simulink model "NL_sin_Park_funciona"  (R2023b)
settings: Solver=VariableStepAuto  StartTime=0.0  StopTime=2  MaxStep=1e-3  RelTol=1e-3
values from neighbouring files (symbols this model uses):
  alpha_Cu = 3.9e-3    (= 0.0039)    [definicion_cte.m]
  b_eq = b_m + b_l/(r^2)    (= 2.40277777778e-05)    [definicion_cte.m]
  C_ts = 0.818    [definicion_cte.m]
  g = 9.80665    [definicion_cte.m]
  J_eq = J_m + J_l/(r^2)    (= 4.58263888889e-05)    [definicion_cte.m]
  k_l = m*l_cm + m_l*l_l    (= 1)    [definicion_cte.m]
  L_d = 6.6e-3    (= 0.0066)    [definicion_cte.m]
  L_ls = 0.8e-3    (= 0.0008)    [definicion_cte.m]
  L_q = 5.8e-3    (= 0.0058)    [definicion_cte.m]
  lambda_m = 0.016    [definicion_cte.m]
  P_p = 3    [definicion_cte.m]
  r = 120    [definicion_cte.m]
  R_sREF = 1.02    [definicion_cte.m]
  R_tsamb = 146.7    [definicion_cte.m]
  T_amb = 25    [definicion_cte.m]
  T_sREF = 20    [definicion_cte.m]
undefined symbols (not defined in the file or in its folder): magnitude
libraries: SignalEditorBlockLib x2
settings Model: Creator=MSI  LastModifiedBy=MSI

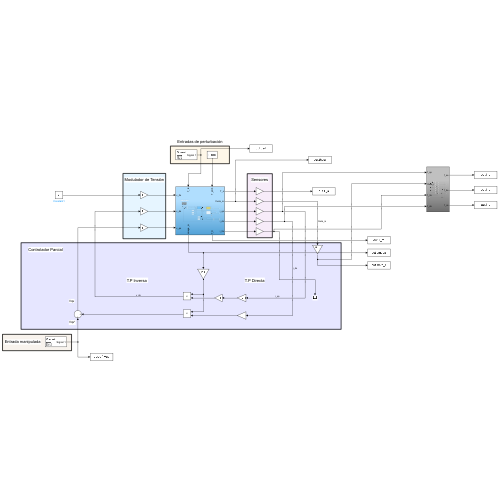
[thumbnail: Simulink's stored preview of the top-level diagram]
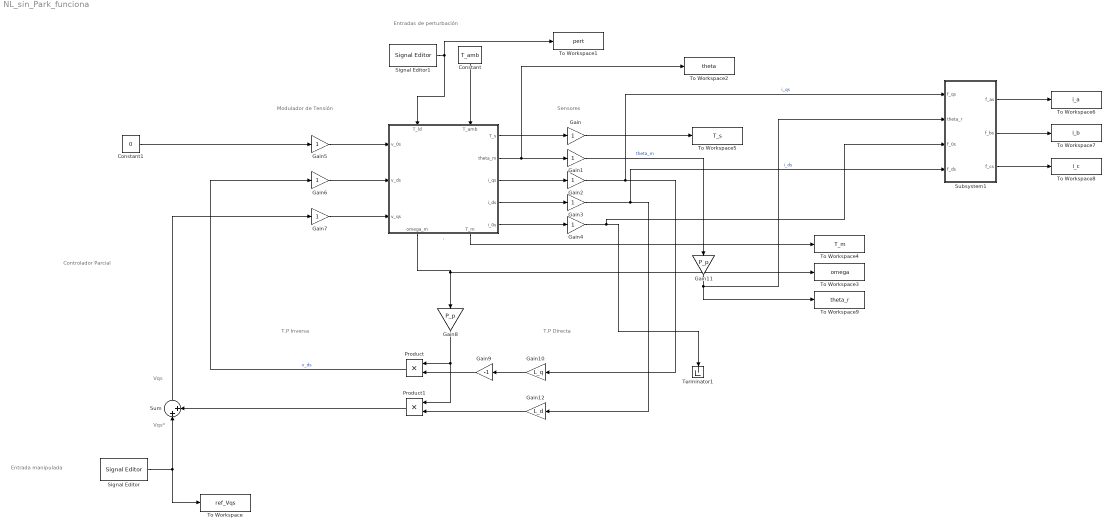
== system NL_sin_Park_funciona ==
  note: T.P Inversa
  note: Vqs
  note: Controlador Parcial
  note: Entrada manipulada
  note: Vqs*
  note: Modulador de Tensión
  note: Sensores
  note: Entradas de perturbación
  note: T.P Directa
  . : Subsystem
      settings: PortSchema="{\"entries\":[{\"content\":{\"sides\":[{\"content\":{\"connectorIds\":[\"In1\",\"In2\",\"In3\"]},\"type\":\"ConnectorPlacement.EquallySpacedRectSide\",\"uuid\":\"a2221977-a2db-4f9f-a6b6-e4e93ab83132\"},{\"content\":{\"connectorIds\":[\"Out1\",\"Out2\",\"Out3\",\"Out4\",\"Out5\"],\"side\":\"RIGHT\"},\"type\":\"ConnectorPlacement.EquallySpacedRectSide\",\"uuid\":\"4d1b64fb-cd5f-444c-9c55-dd968f667727\"},{\"content\":{\"connectorIds\":[\"In4\",\"In5\"],\"side\":\"TOP\"},\"type\":\"ConnectorPlacement.EquallySpacedRectSide\",\"uuid\":\"feec2d7e-2013-4827-9d2d-5413e6a364ce\"},{\"content\":{\"connectorIds\":[\"Out6\",\"Out7\"],\"side\":\"BOTTOM\"},\"type\":\"ConnectorPlacement.EquallySpacedRectSide\",\"uuid\":\"a4e68a75-7272-4a37-88ea-97e0fe693470\"}]},\"type\":\"ConnectorPlacement.EquallySpacedConnector\",\"uuid\":\"3fef7616-1be8-4199-84fe-e5c97ae42ef2\"}],\"packageUris\":[\"http://schema.mathworks.com/mf0/Connector/R2020b\"],\"version\":\"1.0\"}"
  Constant : Constant  Value=T_amb
  Constant1 : Constant  Value=0
  Gain{,1..7} (8 alike) : Gain
  Gain10 : Gain  Gain=L_q
  Gain11 : Gain  Gain=P_p
  Gain12 : Gain  Gain=L_d
  Gain8 : Gain  Gain=P_p
  Gain9 : Gain  Gain=-1
  Product : Product
  Product1 : Product
  Signal Editor : SignalEditorBlockLib/Signal Editor  FileName=Vq.mat  ActiveScenario=Scenario  ActiveSignal=Signal 1  IsBus=off  OutputBusObjectStr=Bus: BusObject  SampleTime=0  Interpolate=off  ZeroCross=off  OutputAfterFinalValue=Setting to zero  Unit=inherit  PreserveSignalName=on  ApplySigPropsToAllScenarios=on  ApplySigPropsToAllSignals=off
  Signal Editor1 : SignalEditorBlockLib/Signal Editor  FileName=C:\Users\MSI\Documents\FING\Materias\AyME\Repo_proyecto\AyME\Avances_Sito\Tl.mat  ActiveScenario=Scenario  ActiveSignal=Signal 1  IsBus=off  OutputBusObjectStr=Bus: BusObject  SampleTime=0  Interpolate=off  ZeroCross=off  OutputAfterFinalValue=Setting to zero  Unit=inherit  PreserveSignalName=on  ApplySigPropsToAllScenarios=on  ApplySigPropsToAllSignals=off
  Subsystem1 : Subsystem
  Sum : Sum  Inputs=|++
  Terminator1 : Terminator
  To Workspace : ToWorkspace  VariableName=ref_Vqs  SaveFormat=Timeseries  SampleTime=-1
  To Workspace1 : ToWorkspace  VariableName=pert  SaveFormat=Timeseries  SampleTime=-1
  To Workspace2 : ToWorkspace  VariableName=theta  SaveFormat=Timeseries  SampleTime=-1
  To Workspace3 : ToWorkspace  VariableName=omega  SaveFormat=Timeseries  SampleTime=-1
  To Workspace4 : ToWorkspace  VariableName=T_m  SaveFormat=Timeseries  SampleTime=-1
  To Workspace5 : ToWorkspace  VariableName=T_s  SaveFormat=Timeseries  SampleTime=-1
  To Workspace6 : ToWorkspace  VariableName=i_a  SaveFormat=Timeseries  SampleTime=-1
  To Workspace7 : ToWorkspace  VariableName=i_b  SaveFormat=Timeseries  SampleTime=-1
  To Workspace8 : ToWorkspace  VariableName=i_c  SaveFormat=Timeseries  SampleTime=-1
  To Workspace9 : ToWorkspace  VariableName=theta_r  SaveFormat=Timeseries  SampleTime=-1
  wires:
  Product1/1 -> Sum/2
  Gain6/1 -> ./2(v_ds)
  Gain7/1 -> ./3(v_qs)
  Gain4/1 -> Subsystem1/3(f_0s), Terminator1/1
  Sum/1 -> Gain7/1
  ./7(T_m) -> To Workspace4/1
  ./1(T_s) -> Gain/1
  ./5(i_0s) -> Gain4/1
  ./4(i_ds) -> Gain3/1
  ./3(i_qs) -> Gain2/1
  Gain9/1 -> Product/2
  Gain5/1 -> ./1(v_0s)
  ./6(omega_m) -> Gain8/1, To Workspace3/1
  Gain3/1 -> Subsystem1/4(f_ds), Gain12/1  "i_ds"
  Gain12/1 -> Product1/2
  Gain2/1 -> Subsystem1/1(f_qs), Gain10/1  "i_qs"
  Gain1/1 -> Gain11/1  "theta_m"
  ./2(theta_m) -> To Workspace2/1, Gain1/1
  Gain11/1 -> Subsystem1/2(theta_r), To Workspace9/1
  Gain10/1 -> Gain9/1
  Signal Editor/1 -> To Workspace/1, Sum/1
  Gain/1 -> To Workspace5/1
  Gain8/1 -> Product1/1, Product/1
  Signal Editor1/1 -> To Workspace1/1, ./4(T_ld)
  Product/1 -> Gain6/1  "v_ds"
  Constant1/1 -> Gain5/1
  Constant/1 -> ./5(T_amb)
  Subsystem1/1(f_as) -> To Workspace6/1
  Subsystem1/2(f_bs) -> To Workspace7/1
  Subsystem1/3(f_cs) -> To Workspace8/1

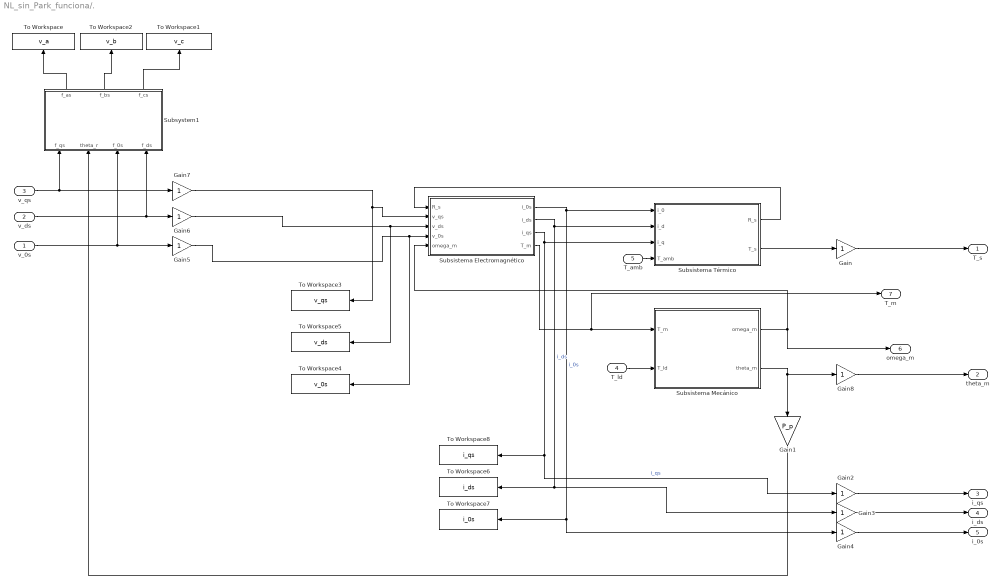
== system NL_sin_Park_funciona/. ==
  v_0s : Inport
  v_ds : Inport  Port=2
  v_qs : Inport  Port=3
  T_ld : Inport  Port=4
  T_amb : Inport  Port=5
  Gain{,2..8} (8 alike) : Gain
  Gain1 : Gain  Gain=P_p
  Subsistema Electromagnético : Subsystem
  Subsistema Mecánico : Subsystem
  Subsistema Térmico : Subsystem
  Subsystem1 : Subsystem
  To Workspace : ToWorkspace  VariableName=v_a  SaveFormat=Timeseries  SampleTime=-1
  To Workspace1 : ToWorkspace  VariableName=v_c  SaveFormat=Timeseries  SampleTime=-1
  To Workspace2 : ToWorkspace  VariableName=v_b  SaveFormat=Timeseries  SampleTime=-1
  To Workspace3 : ToWorkspace  VariableName=v_qs  SaveFormat=Timeseries  SampleTime=-1
  To Workspace4 : ToWorkspace  VariableName=v_0s  SaveFormat=Timeseries  SampleTime=-1
  To Workspace5 : ToWorkspace  VariableName=v_ds  SaveFormat=Timeseries  SampleTime=-1
  To Workspace6 : ToWorkspace  VariableName=i_ds  SaveFormat=Timeseries  SampleTime=-1
  To Workspace7 : ToWorkspace  VariableName=i_0s  SaveFormat=Timeseries  SampleTime=-1
  To Workspace8 : ToWorkspace  VariableName=i_qs  SaveFormat=Timeseries  SampleTime=-1
  T_s : Outport
  theta_m : Outport  Port=2
  i_qs : Outport  Port=3
  i_ds : Outport  Port=4
  i_0s : Outport  Port=5
  omega_m : Outport  Port=6
  T_m : Outport  Port=7
  wires:
  Subsistema Térmico/1(R_s) -> Subsistema Electromagnético/1(R_s)
  Gain7/1 -> To Workspace3/1, Subsistema Electromagnético/2(v_qs)
  Subsistema Mecánico/1(omega_m) -> omega_m/1, Subsistema Electromagnético/5(omega_m)
  Subsistema Electromagnético/1(i_0s) -> Subsistema Térmico/1(i_0), Gain4/1, To Workspace7/1  "i_0s"
  Subsistema Mecánico/2(theta_m) -> Gain1/1, Gain8/1
  Subsistema Electromagnético/4(T_m) -> T_m/1, Subsistema Mecánico/1(T_m)
  Gain3/1 -> i_ds/1
  Subsistema Electromagnético/2(i_ds) -> To Workspace6/1, Gain3/1, Subsistema Térmico/2(i_d)  "i_ds"
  Gain2/1 -> i_qs/1
  T_amb/1 -> Subsistema Térmico/4(T_amb)
  v_ds/1 -> Subsystem1/4(f_ds), Gain6/1
  v_qs/1 -> Subsystem1/1(f_qs), Gain7/1
  v_0s/1 -> Subsystem1/3(f_0s), Gain5/1
  Subsistema Térmico/2(T_s) -> Gain/1
  Subsistema Electromagnético/3(i_qs) -> To Workspace8/1, Gain2/1, Subsistema Térmico/3(i_q)  "i_qs"
  Gain4/1 -> i_0s/1
  Gain5/1 -> To Workspace4/1, Subsistema Electromagnético/4(v_0s)
  T_ld/1 -> Subsistema Mecánico/2(T_ld)
  Gain8/1 -> theta_m/1
  Gain/1 -> T_s/1
  Gain1/1 -> Subsystem1/2(theta_r)
  Gain6/1 -> To Workspace5/1, Subsistema Electromagnético/3(v_ds)
  Subsystem1/1(f_as) -> To Workspace/1
  Subsystem1/2(f_bs) -> To Workspace2/1
  Subsystem1/3(f_cs) -> To Workspace1/1

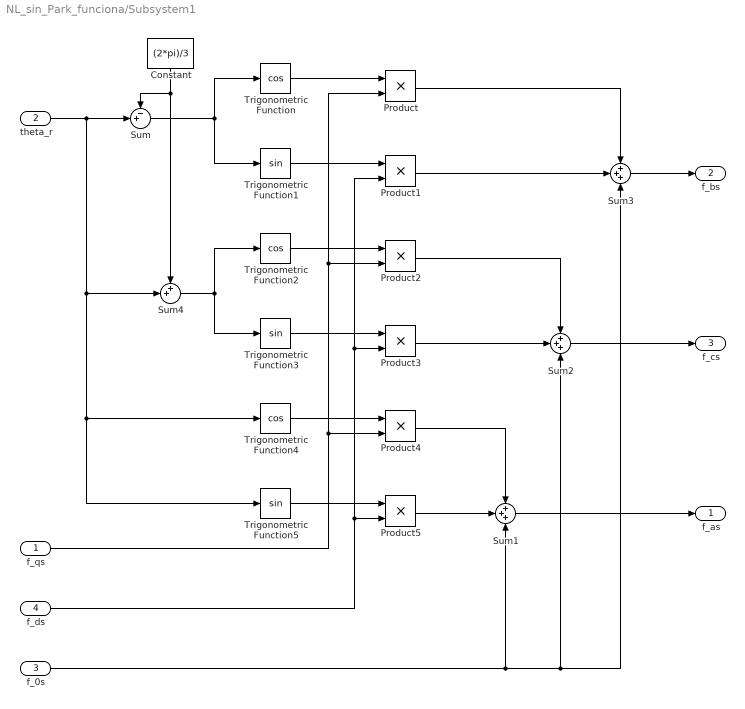
== system NL_sin_Park_funciona/Subsystem1 ==
  f_qs : Inport
  theta_r : Inport  Port=2
  f_0s : Inport  Port=3
  f_ds : Inport  Port=4
  Constant : Constant  Value=(2*pi)/3
  Product{,1..5} (6 alike) : Product
  Sum : Sum  Inputs=-+|
  Sum1 : Sum  Inputs=+++
  Sum2 : Sum  Inputs=+++
  Sum3 : Sum  Inputs=+++
  Sum4 : Sum  Inputs=++|
  Trigonometric Function : Trigonometry  Operator=cos
  Trigonometric Function1 : Trigonometry
  Trigonometric Function2 : Trigonometry  Operator=cos
  Trigonometric Function3 : Trigonometry
  Trigonometric Function4 : Trigonometry  Operator=cos
  Trigonometric Function5 : Trigonometry
  f_as : Outport
  f_bs : Outport  Port=2
  f_cs : Outport  Port=3
  wires:
  Sum1/1 -> f_as/1
  Product5/1 -> Sum1/2
  Sum2/1 -> f_cs/1
  Product1/1 -> Sum3/2
  Trigonometric Function5/1 -> Product5/1
  Sum/1 -> Trigonometric Function1/1, Trigonometric Function/1
  Product2/1 -> Sum2/1
  Product4/1 -> Sum1/1
  f_qs/1 -> Product4/2, Product2/2, Product/2
  Product/1 -> Sum3/1
  f_0s/1 -> Sum3/3, Sum2/3, Sum1/3
  Trigonometric Function4/1 -> Product4/1
  Constant/1 -> Sum4/1, Sum/1
  Trigonometric Function2/1 -> Product2/1
  f_ds/1 -> Product5/2, Product3/2, Product1/2
  Trigonometric Function3/1 -> Product3/1
  Trigonometric Function1/1 -> Product1/1
  Sum4/1 -> Trigonometric Function3/1, Trigonometric Function2/1
  Sum3/1 -> f_bs/1
  theta_r/1 -> Sum4/2, Trigonometric Function5/1, Trigonometric Function4/1, Sum/2
  Product3/1 -> Sum2/2
  Trigonometric Function/1 -> Product/1

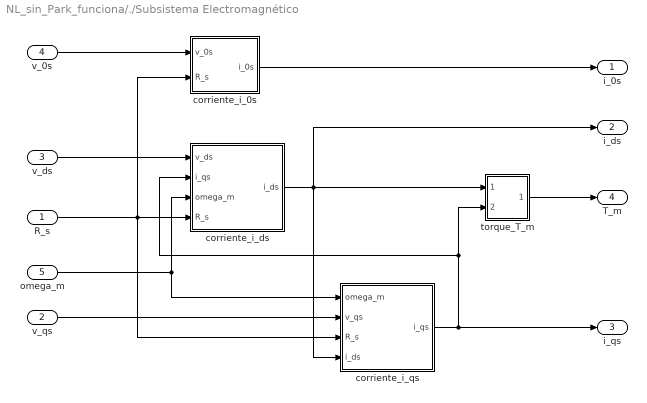
== system NL_sin_Park_funciona/./Subsistema Electromagnético ==
  R_s : Inport
  v_qs : Inport  Port=2
  v_ds : Inport  Port=3
  v_0s : Inport  Port=4
  omega_m : Inport  Port=5
  corriente_i_0s : Subsystem
  corriente_i_ds : Subsystem
  corriente_i_qs : Subsystem
  torque_T_m : Subsystem
  i_0s : Outport
  i_ds : Outport  Port=2
  i_qs : Outport  Port=3
  T_m : Outport  Port=4
  wires:
  R_s/1 -> corriente_i_qs/3(R_s), corriente_i_ds/4(R_s), corriente_i_0s/2(R_s)
  corriente_i_0s/1(i_0s) -> i_0s/1
  corriente_i_qs/1(i_qs) -> i_qs/1, torque_T_m/2(i_qs), corriente_i_ds/2(i_qs)
  corriente_i_ds/1(i_ds) -> corriente_i_qs/4(i_ds), torque_T_m/1(i_ds), i_ds/1
  v_0s/1 -> corriente_i_0s/1(v_0s)
  v_ds/1 -> corriente_i_ds/1(v_ds)
  omega_m/1 -> corriente_i_qs/1(omega_m), corriente_i_ds/3(omega_m)
  v_qs/1 -> corriente_i_qs/2(v_qs)
  torque_T_m/1(T_m) -> T_m/1

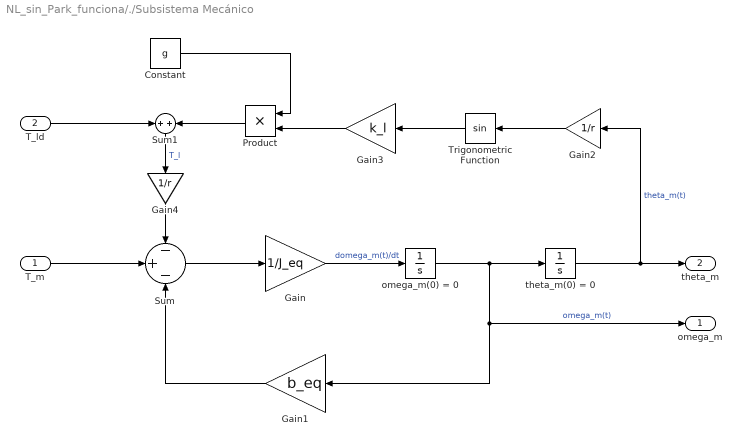
== system NL_sin_Park_funciona/./Subsistema Mecánico ==
  T_m : Inport
  T_ld : Inport  Port=2
  Constant : Constant  Value=g
  Gain : Gain  Gain=1/J_eq
  Gain1 : Gain  Gain=b_eq
  Gain2 : Gain  Gain=1/r
  Gain3 : Gain  Gain=k_l
  Gain4 : Gain  Gain=1/r
  Product : Product
  Sum : Sum  Inputs=-+-
  Sum1 : Sum
  Trigonometric Function : Trigonometry
  "omega_m(0) = 0\t" : Integrator
  theta_m(0) = 0 : Integrator
  omega_m : Outport
  theta_m : Outport  Port=2
  wires:
  Product/1 -> Sum1/2
  Constant/1 -> Product/1
  T_m/1 -> Sum/2
  Gain3/1 -> Product/2
  T_ld/1 -> Sum1/1
  Gain1/1 -> Sum/3
  Gain4/1 -> Sum/1
  Sum1/1 -> Gain4/1  "T_l"
  theta_m(0) = 0/1 -> Gain2/1, theta_m/1  "theta_m(t)"
  Trigonometric Function/1 -> Gain3/1
  Sum/1 -> Gain/1
  Gain2/1 -> Trigonometric Function/1
  "omega_m(0) = 0\t"/1 -> theta_m(0) = 0/1, omega_m/1, Gain1/1  "omega_m(t)"
  Gain/1 -> "omega_m(0) = 0\t"/1  "domega_m(t)/dt"

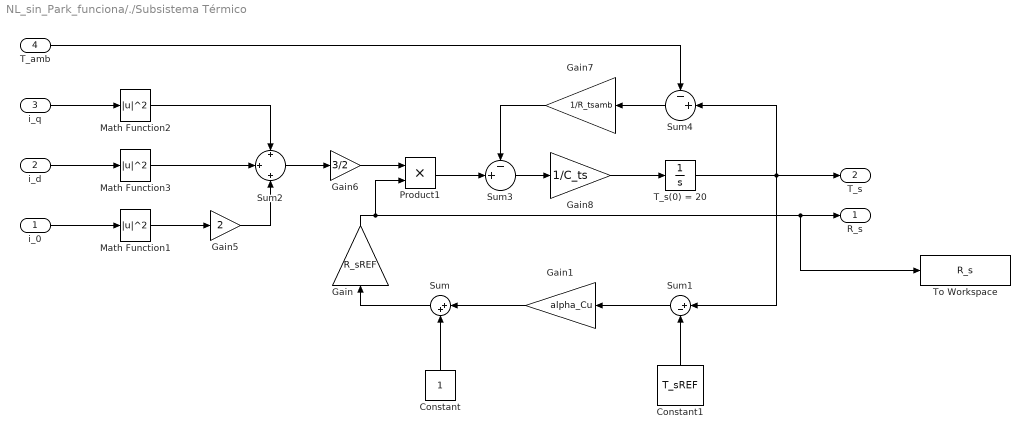
== system NL_sin_Park_funciona/./Subsistema Térmico ==
  i_0 : Inport
  i_d : Inport  Port=2
  i_q : Inport  Port=3
  T_amb : Inport  Port=4
  Constant : Constant
  Constant1 : Constant  Value=T_sREF
  Gain : Gain  Gain=R_sREF
  Gain1 : Gain  Gain=alpha_Cu
  Gain5 : Gain  Gain=2
  Gain6 : Gain  Gain=3/2
  Gain7 : Gain  Gain=1/R_tsamb
  Gain8 : Gain  Gain=1/C_ts
  Math Function1 : Math  Operator=magnitude^2  OutputSignalType=real
  Math Function2 : Math  Operator=magnitude^2  OutputSignalType=real
  Math Function3 : Math  Operator=magnitude^2  OutputSignalType=real
  Product1 : Product
  Sum : Sum  Inputs=|++
  Sum1 : Sum  Inputs=|+-
  Sum2 : Sum  Inputs=+|+|+
  Sum3 : Sum  Inputs=-+|
  Sum4 : Sum  Inputs=-+|
  T_s(0) = 20 : Integrator  InitialCondition=20
  To Workspace : ToWorkspace  VariableName=R_s  SaveFormat=Timeseries  SampleTime=-1
  R_s : Outport
  T_s : Outport  Port=2
  wires:
  i_q/1 -> Math Function2/1
  i_d/1 -> Math Function3/1
  i_0/1 -> Math Function1/1
  Gain1/1 -> Sum/1
  Gain8/1 -> T_s(0) = 20/1
  Sum3/1 -> Gain8/1
  Constant/1 -> Sum/2
  Product1/1 -> Sum3/2
  Sum/1 -> Gain/1
  T_amb/1 -> Sum4/1
  Math Function1/1 -> Gain5/1
  Sum4/1 -> Gain7/1
  T_s(0) = 20/1 -> Sum1/1, Sum4/2, T_s/1
  Sum2/1 -> Gain6/1
  Sum1/1 -> Gain1/1
  Gain6/1 -> Product1/1
  Constant1/1 -> Sum1/2
  Gain5/1 -> Sum2/3
  Gain7/1 -> Sum3/1
  Math Function2/1 -> Sum2/1
  Math Function3/1 -> Sum2/2
  Gain/1 -> To Workspace/1, R_s/1, Product1/2

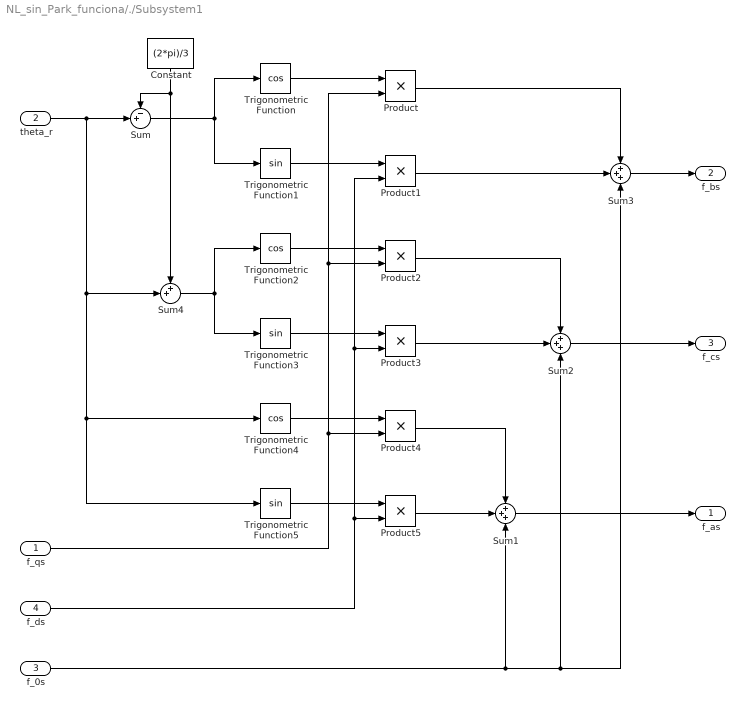
== system NL_sin_Park_funciona/./Subsystem1 ==
  f_qs : Inport
  theta_r : Inport  Port=2
  f_0s : Inport  Port=3
  f_ds : Inport  Port=4
  Constant : Constant  Value=(2*pi)/3
  Product{,1..5} (6 alike) : Product
  Sum : Sum  Inputs=-+|
  Sum1 : Sum  Inputs=+++
  Sum2 : Sum  Inputs=+++
  Sum3 : Sum  Inputs=+++
  Sum4 : Sum  Inputs=++|
  Trigonometric Function : Trigonometry  Operator=cos
  Trigonometric Function1 : Trigonometry
  Trigonometric Function2 : Trigonometry  Operator=cos
  Trigonometric Function3 : Trigonometry
  Trigonometric Function4 : Trigonometry  Operator=cos
  Trigonometric Function5 : Trigonometry
  f_as : Outport
  f_bs : Outport  Port=2
  f_cs : Outport  Port=3
  wires:
  Sum1/1 -> f_as/1
  Product5/1 -> Sum1/2
  Sum2/1 -> f_cs/1
  Product1/1 -> Sum3/2
  Trigonometric Function5/1 -> Product5/1
  Sum/1 -> Trigonometric Function1/1, Trigonometric Function/1
  Product2/1 -> Sum2/1
  Product4/1 -> Sum1/1
  f_qs/1 -> Product4/2, Product2/2, Product/2
  Product/1 -> Sum3/1
  f_0s/1 -> Sum3/3, Sum2/3, Sum1/3
  Trigonometric Function4/1 -> Product4/1
  Constant/1 -> Sum4/1, Sum/1
  Trigonometric Function2/1 -> Product2/1
  f_ds/1 -> Product5/2, Product3/2, Product1/2
  Trigonometric Function3/1 -> Product3/1
  Trigonometric Function1/1 -> Product1/1
  Sum4/1 -> Trigonometric Function3/1, Trigonometric Function2/1
  Sum3/1 -> f_bs/1
  theta_r/1 -> Sum4/2, Trigonometric Function5/1, Trigonometric Function4/1, Sum/2
  Product3/1 -> Sum2/2
  Trigonometric Function/1 -> Product/1

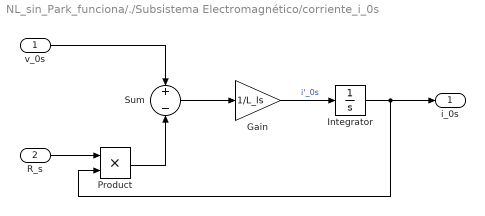
== system NL_sin_Park_funciona/./Subsistema Electromagnético/corriente_i_0s ==
  v_0s : Inport
  R_s : Inport  Port=2
  Gain : Gain  Gain=1/L_ls
  Integrator : Integrator
  Product : Product
  Sum : Sum  Inputs=+-
  i_0s : Outport
  wires:
  Sum/1 -> Gain/1
  Gain/1 -> Integrator/1  "i'_0s"
  Integrator/1 -> i_0s/1, Product/2
  Product/1 -> Sum/2
  v_0s/1 -> Sum/1
  R_s/1 -> Product/1

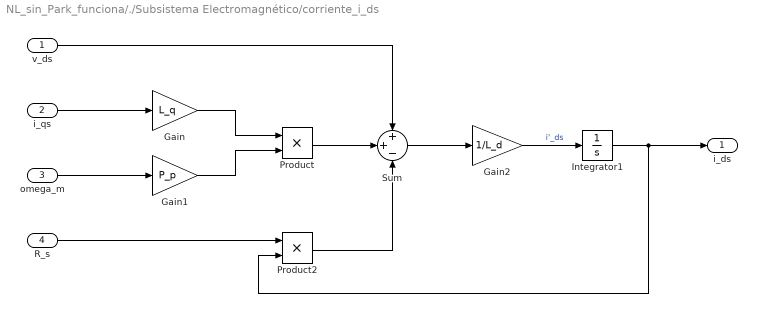
== system NL_sin_Park_funciona/./Subsistema Electromagnético/corriente_i_ds ==
  v_ds : Inport
  i_qs : Inport  Port=2
  omega_m : Inport  Port=3
  R_s : Inport  Port=4
  Gain : Gain  Gain=L_q
  Gain1 : Gain  Gain=P_p
  Gain2 : Gain  Gain=1/L_d
  Integrator1 : Integrator
  Product : Product
  Product2 : Product
  Sum : Sum  Inputs=++-
  i_ds : Outport
  wires:
  Gain1/1 -> Product/2
  Gain/1 -> Product/1
  i_qs/1 -> Gain/1
  Product/1 -> Sum/2
  Integrator1/1 -> i_ds/1, Product2/2
  v_ds/1 -> Sum/1
  Gain2/1 -> Integrator1/1  "i'_ds"
  R_s/1 -> Product2/1
  Sum/1 -> Gain2/1
  Product2/1 -> Sum/3
  omega_m/1 -> Gain1/1

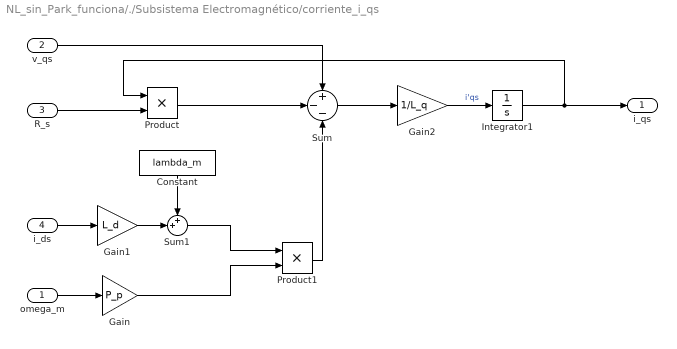
== system NL_sin_Park_funciona/./Subsistema Electromagnético/corriente_i_qs ==
  omega_m : Inport
  v_qs : Inport  Port=2
  R_s : Inport  Port=3
  i_ds : Inport  Port=4
  Constant : Constant  Value=lambda_m
  Gain : Gain  Gain=P_p
  Gain1 : Gain  Gain=L_d
  Gain2 : Gain  Gain=1/L_q
  Integrator1 : Integrator
  Product : Product
  Product1 : Product
  Sum : Sum  Inputs=+--
  Sum1 : Sum  Inputs=++|
  i_qs : Outport
  wires:
  Gain1/1 -> Sum1/2
  Product/1 -> Sum/2
  R_s/1 -> Product/2
  Sum1/1 -> Product1/1
  v_qs/1 -> Sum/1
  Gain/1 -> Product1/2
  Gain2/1 -> Integrator1/1  "i'qs"
  Constant/1 -> Sum1/1
  i_ds/1 -> Gain1/1
  Sum/1 -> Gain2/1
  omega_m/1 -> Gain/1
  Integrator1/1 -> i_qs/1, Product/1
  Product1/1 -> Sum/3

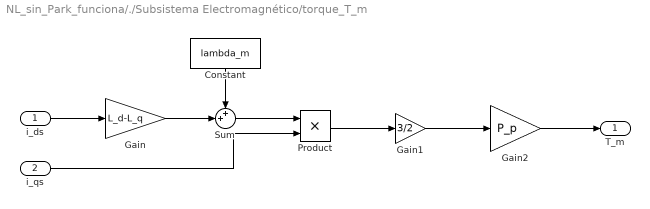
== system NL_sin_Park_funciona/./Subsistema Electromagnético/torque_T_m ==
  i_ds : Inport
  i_qs : Inport  Port=2
  Constant : Constant  Value=lambda_m
  Gain : Gain  Gain=L_d-L_q
  Gain1 : Gain  Gain=3/2
  Gain2 : Gain  Gain=P_p
  Product : Product
  Sum : Sum  Inputs=++|
  T_m : Outport
  wires:
  Constant/1 -> Sum/1
  Gain/1 -> Sum/2
  i_ds/1 -> Gain/1
  Product/1 -> Gain1/1
  i_qs/1 -> Product/2
  Sum/1 -> Product/1
  Gain1/1 -> Gain2/1
  Gain2/1 -> T_m/1
